simulink model "model1"  (R2017a)
settings: Solver=VariableStepAuto  StartTime=0.0  StopTime=10.0  RelTol=1e-3
settings Model: Creator=Peter Vanhoef  LastModifiedBy=Peter Vanhoef

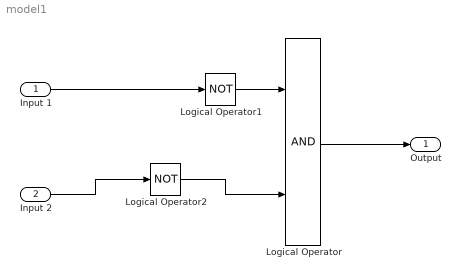
== system model1 ==
  Input 1 : Inport
  Input 2 : Inport  Port=2
  Logical Operator : Logic  AllPortsSameDT=off  OutDataTypeStr=boolean
  Logical Operator1 : Logic  Operator=NOT  Inputs=1  AllPortsSameDT=off  OutDataTypeStr=boolean
  Logical Operator2 : Logic  Operator=NOT  AllPortsSameDT=off  OutDataTypeStr=boolean
  Output : Outport
  wires:
  Input 1/1 -> Logical Operator1/1
  Logical Operator/1 -> Output/1
  Logical Operator1/1 -> Logical Operator/1
  Input 2/1 -> Logical Operator2/1
  Logical Operator2/1 -> Logical Operator/2
